simulink model "simulink"  (R2024b)
settings: Solver=ode4  StartTime=0.0  StopTime=60  FixedStep=0.005  MaxStep=0.01  MinStep=1e-06  RelTol=1e-3
values from neighbouring files (symbols this model uses):
  Cd = 0.36    [main.m]
  Cr = 0.01    [main.m]
  gear_ratio = 5    [main.m]
  initial_velocity = 0    [main.m]
  max_brake_torque = 20000    [main.m]
  track_x = track_x(:)    [main.m]    (also in plotRaceTrack.m = [x1, x2, x3, x4])
  track_y = track_y(:)    [main.m]    (also in plotRaceTrack.m = [y1, y2, y3, y4])
  v_des_straight = 15    [main.m]
  v_des_turn = 10    [main.m]
undefined symbols (not defined in the file or in its folder): carData, datBat, datMotor
libraries: slpidlib x2
settings Model: Creator=gavin  LastModifiedBy=sharj
settings SolverCC: InitialStep=1e-06

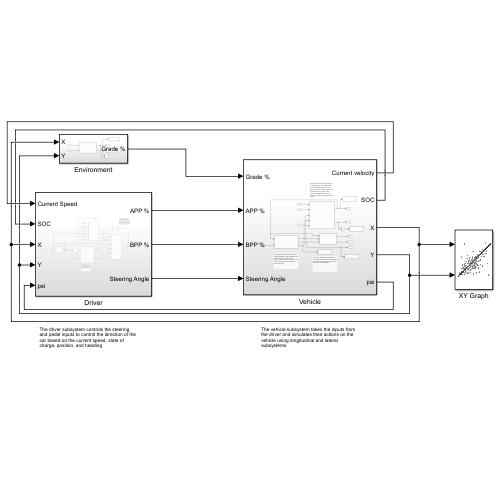
[thumbnail: Simulink's stored preview of the top-level diagram]
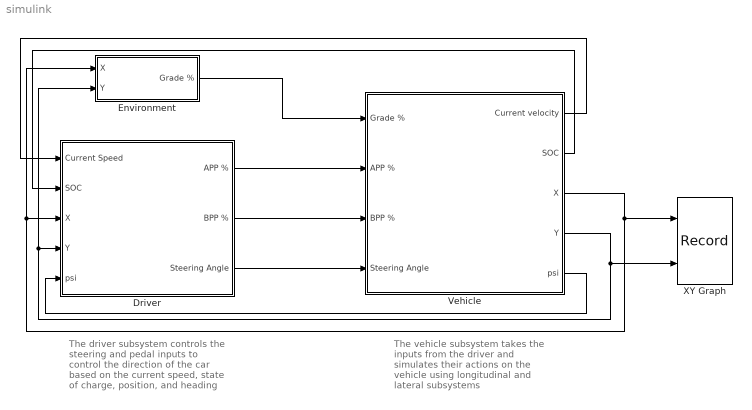
== system simulink ==
  note: The driver subsystem controls the steering and pedal inputs to control the direction of the car based on the current speed, state of charge, position, and heading
  note: The vehicle subsystem takes the inputs from the driver and simulates their actions on the vehicle using longitudinal and lateral subsystems
  Driver : Subsystem
  Environment : Subsystem
  Vehicle : Subsystem
  XY Graph : Record  FileSettingsInternal="{\"entries\":[{\"content\":{\"excelSettings\":{\"content\":{},\"type\":\"Streamout.ExcelSettings\"}},\"type\":\"Streamout.FileSettingStorage\",\"uuid\":\"\"}],\"packageUris\":[\"http:\\/\\/schema.mathworks.com\\/mf0\\/streamout_blocks\\/R2020a\"],\"version\":\"1.0\"}"  Layout=[1 1]  SignalsInternal="{\"entries\":[{\"content\":{\"signals\":[{\"content\":{\"blockPath\":[],\"dimensions\":[1],\"domain\":\"\",\"lineColor\":\"#a2142f\",\"plots\":[ 1 ],\"port\":1,\"signalID\":1,\"signalName\":\"Vehicle:3\"},\"type\":\"RecordBlkView.Signal\",\"uuid\":\"\"},{\"content\":{\"blockPath\":[],\"dimensions\":[1],\"domain\":\"\",\"lineColor\":\"#139fff\",\"plots\":[ 1 ],\"port\":2,\"signalID\":2,\"signalName\":\"Vehicle:4\"},\"type\":\"RecordBlkView.Signal\",\"uuid\":\"\"}]},\"type\":\"RecordBlkView.InputSignals\",\"uuid\":\"\"}],\"packageUris\":[\"http:\\/\\/schema.mathworks.com\\/mf0\\/streamout_blocks\\/R2020a\"],\"version\":\"1.0\"}"  VisualizationBindings="{\"xyplotplugin\":{\"info\":[{\"series\":[{\"bindingParametersList\":[{\"parameter\":\"X-Axis\",\"signalID\":1,\"signalName\":\"Vehicle:3\"},{\"parameter\":\"Y-Axis\",\"signalID\":2,\"signalName\":\"Vehicle:4\"}],\"seriesID\":0}],\"subplotID\":1}]}}"  CompatibilityTag=XY
  wires:
  Vehicle/3(X) -> XY Graph/1, Environment/1(X), Driver/3(X)
  Vehicle/4(Y) -> Environment/2(Y), Driver/4(Y), XY Graph/2
  Driver/1(APP %) -> Vehicle/2(APP %)
  Driver/2(BPP %) -> Vehicle/3(BPP %)
  Driver/3(Steering Angle) -> Vehicle/4(Steering Angle)
  Environment/1(Grade %) -> Vehicle/1(Grade %)
  Vehicle/2(SOC) -> Driver/2(SOC)
  Vehicle/1(Current velocity) -> Driver/1(Current Speed)
  Vehicle/5(psi) -> Driver/5(psi)

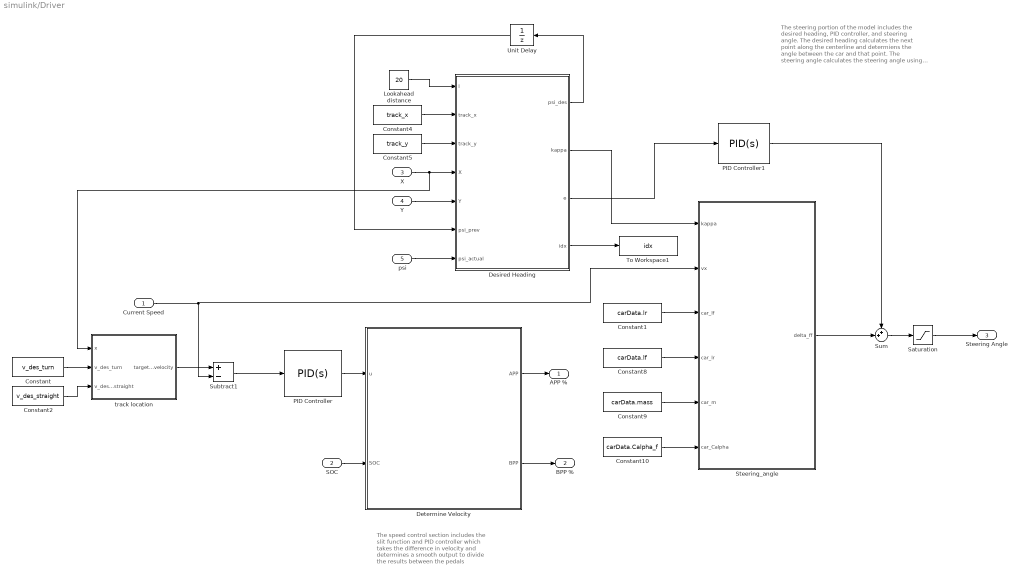
== system simulink/Driver ==
  note: The speed control section includes the slit function and PID controller which takes the difference in velocity and determines a smooth output to divide the results between the pedals
  note: The steering portion of the model includes the desired heading, PID controller, and steering angle. The desired heading calculates the next point along the centerline and determiens the angle between the car and that point. The steering angle calculates the steering angle using the feed forward method. The PID controller smooths the results and provides feedback to ensure resilience to small changes in the system.
  Current Speed : Inport
  SOC : Inport  Port=2
  X : Inport  Port=3
  Y : Inport  Port=4
  psi : Inport  Port=5
  Constant : Constant  Value=v_des_turn
  Constant1 : Constant  Value=carData.lr
  Constant10 : Constant  Value=carData.Calpha_f
  Constant2 : Constant  Value=v_des_straight
  Constant4 : Constant  Value=track_x
  Constant5 : Constant  Value=track_y
  Constant8 : Constant  Value=carData.lf
  Constant9 : Constant  Value=carData.mass
  Desired Heading : MATLAB Function  TreatAsAtomicUnit=on
  Determine Velocity : MATLAB Function  TreatAsAtomicUnit=on
  Lookahead distance : Constant  Value=20
  PID Controller : slpidlib/PID Controller  Controller=PID  Form=Parallel  TimeDomain=Continuous-time  UseExternalTs=off  SampleTime=-1  IntegratorMethod=Forward Euler  FilterMethod=Forward Euler  ControllerParametersSource=internal  P=0.9  I=0.2  UseKiTs=off  D=0  UseExternalDerivativeSource=off  N=100  UseFilter=on  TunerSelectOption=Transfer Function Based (PID Tuner App)  InitialConditionSource=internal  InitialConditionForIntegrator=0  InitialConditionForFilter=0  DifferentiatorICPrevScaledInput=0  ExternalReset=none  TrackingMode=off  Kt=1  LimitOutput=on  SatLimitsSource=internal  UpperSaturationLimit=1  LowerSaturationLimit=-1  LinearizeAsGain=on  AntiWindupMode=none  Kb=1  LimitIntegrator=off  UpperIntegratorSaturationLimit=inf  LowerIntegratorSaturationLimit=-inf  POutMin=[]  POutMax=[]  IOutMin=[]  IOutMax=[]  DOutMin=[]  DOutMax=[]  NOutMin=[]  NOutMax=[]  SumOutMin=[]  SumOutMax=[]  SaturationOutMin=[]  SaturationOutMax=[]  PParamMin=[]  PParamMax=[]  IParamMin=[]  IParamMax=[]  DParamMin=[]  DParamMax=[]  NParamMin=[]  NParamMax=[]  KbParamMin=[]  KbParamMax=[]  KtParamMin=[]  KtParamMax=[]  KbOutMin=[]  KbOutMax=[]  KtOutMin=[]  KtOutMax=[]  IntegratorOutMin=[]  IntegratorOutMax=[]  FilterOutMin=[]  FilterOutMax=[]  SumI1OutMin=[]  SumI1OutMax=[]  SumI2OutMin=[]  SumI2OutMax=[]  SumI3OutMin=[]  SumI3OutMax=[]  SumI4OutMin=[]  SumI4OutMax=[]  SumDOutMin=[]  SumDOutMax=[]  DifferentiatorOutMin=[]  DifferentiatorOutMax=[]  FilterDiffOutCoefMin=[]  FilterDiffOutCoefMax=[]  ReciprocalOutMin=[]  ReciprocalOutMax=[]  SumDenOutMin=[]  SumDenOutMax=[]  SumNumOutMin=[]  SumNumOutMax=[]  DivideOutMin=[]  DivideOutMax=[]  UdiffTsProdOutMin=[]  UdiffTsProdOutMax=[]  NTsProdOutMin=[]  NTsProdOutMax=[]  UintegralTsProdOutMin=[]  UintegralTsProdOutMax=[]  UngainTsProdOutMin=[]  UngainTsProdOutMax=[]  ClampingZeroOutDataTypeStr=Inherit: Inherit via back propagation  ClampingZeroOutMin=[]  ClampingZeroOutMax=[]  FilterDenConstantOutDataTypeStr=Inherit: Inherit via back propagation  FilterDenConstantOutMin=[]  FilterDenConstantOutMax=[]  PCopyOutDataTypeStr=Inherit: Inherit via back propagation  PCopyOutMin=[]  PCopyOutMax=[]  NCopyOutDataTypeStr=Inherit: Inherit via back propagation  NCopyOutMin=[]  NCopyOutMax=[]  IntegratorContinuousStateAttributes=''  IntegratorStateMustResolveToSignalObject=off  IntegratorRTWStateStorageClass=Auto  FilterContinuousStateAttributes=''  FilterStateMustResolveToSignalObject=off  FilterRTWStateStorageClass=Auto  ParallelPVariant=InternalParameters  IdealPVariant=Disabled  IVariant=InternalParameters  DVariant=InternalParameters  IntegratorVariant=Continuous  SatVariant=Disabled  AWVariant=Passthrough  PCopyVariant=Disabled  TRVariant=Disabled  FdbkBlocksVariant=Forward  IdealPFdbkVariant=Disabled  SatFdbkVariant=Disabled  DerivativeFilterVariant=ContFilter  NVariant=InternalParameters  NCopyVariant=Disabled  FilterICVariant=InternalICsFilter  IntegratorICVariant=InternalICs  ExternalResetVariant=Disabled  TRSumVariant=Passthrough  SumFdbkVariant=Disabled  SumVariant=Sum_PID  TsampFilterVariant=InternalTs  TsampNgainVariant=Passthrough  TsampIntegralVariant=Passthrough  ExternalSaturationOutDataTypeStr=Inherit: Same as second input  DerivativeSourceVariant=ErrorSignal  PreIntVariant=InternalPreInt
  PID Controller1 : slpidlib/PID Controller  Controller=PID  Form=Parallel  TimeDomain=Continuous-time  UseExternalTs=off  SampleTime=-1  IntegratorMethod=Forward Euler  FilterMethod=Forward Euler  ControllerParametersSource=internal  P=1  I=1  UseKiTs=off  D=0  UseExternalDerivativeSource=off  N=100  UseFilter=on  TunerSelectOption=Transfer Function Based (PID Tuner App)  InitialConditionSource=internal  InitialConditionForIntegrator=0  InitialConditionForFilter=0  DifferentiatorICPrevScaledInput=0  ExternalReset=none  TrackingMode=off  Kt=1  LimitOutput=off  SatLimitsSource=internal  UpperSaturationLimit=inf  LowerSaturationLimit=-inf  LinearizeAsGain=on  AntiWindupMode=none  Kb=1  LimitIntegrator=off  UpperIntegratorSaturationLimit=inf  LowerIntegratorSaturationLimit=-inf  POutMin=[]  POutMax=[]  IOutMin=[]  IOutMax=[]  DOutMin=[]  DOutMax=[]  NOutMin=[]  NOutMax=[]  SumOutMin=[]  SumOutMax=[]  SaturationOutMin=[]  SaturationOutMax=[]  PParamMin=[]  PParamMax=[]  IParamMin=[]  IParamMax=[]  DParamMin=[]  DParamMax=[]  NParamMin=[]  NParamMax=[]  KbParamMin=[]  KbParamMax=[]  KtParamMin=[]  KtParamMax=[]  KbOutMin=[]  KbOutMax=[]  KtOutMin=[]  KtOutMax=[]  IntegratorOutMin=[]  IntegratorOutMax=[]  FilterOutMin=[]  FilterOutMax=[]  SumI1OutMin=[]  SumI1OutMax=[]  SumI2OutMin=[]  SumI2OutMax=[]  SumI3OutMin=[]  SumI3OutMax=[]  SumI4OutMin=[]  SumI4OutMax=[]  SumDOutMin=[]  SumDOutMax=[]  DifferentiatorOutMin=[]  DifferentiatorOutMax=[]  FilterDiffOutCoefMin=[]  FilterDiffOutCoefMax=[]  ReciprocalOutMin=[]  ReciprocalOutMax=[]  SumDenOutMin=[]  SumDenOutMax=[]  SumNumOutMin=[]  SumNumOutMax=[]  DivideOutMin=[]  DivideOutMax=[]  UdiffTsProdOutMin=[]  UdiffTsProdOutMax=[]  NTsProdOutMin=[]  NTsProdOutMax=[]  UintegralTsProdOutMin=[]  UintegralTsProdOutMax=[]  UngainTsProdOutMin=[]  UngainTsProdOutMax=[]  ClampingZeroOutDataTypeStr=Inherit: Inherit via back propagation  ClampingZeroOutMin=[]  ClampingZeroOutMax=[]  FilterDenConstantOutDataTypeStr=Inherit: Inherit via back propagation  FilterDenConstantOutMin=[]  FilterDenConstantOutMax=[]  PCopyOutDataTypeStr=Inherit: Inherit via back propagation  PCopyOutMin=[]  PCopyOutMax=[]  NCopyOutDataTypeStr=Inherit: Inherit via back propagation  NCopyOutMin=[]  NCopyOutMax=[]  IntegratorContinuousStateAttributes=''  IntegratorStateMustResolveToSignalObject=off  IntegratorRTWStateStorageClass=Auto  FilterContinuousStateAttributes=''  FilterStateMustResolveToSignalObject=off  FilterRTWStateStorageClass=Auto  ParallelPVariant=InternalParameters  IdealPVariant=Disabled  IVariant=InternalParameters  DVariant=InternalParameters  IntegratorVariant=Continuous  SatVariant=Disabled  AWVariant=Passthrough  PCopyVariant=Disabled  TRVariant=Disabled  FdbkBlocksVariant=Forward  IdealPFdbkVariant=Disabled  SatFdbkVariant=Disabled  DerivativeFilterVariant=ContFilter  NVariant=InternalParameters  NCopyVariant=Disabled  FilterICVariant=InternalICsFilter  IntegratorICVariant=InternalICs  ExternalResetVariant=Disabled  TRSumVariant=Passthrough  SumFdbkVariant=Disabled  SumVariant=Sum_PID  TsampFilterVariant=InternalTs  TsampNgainVariant=Passthrough  TsampIntegralVariant=Passthrough  ExternalSaturationOutDataTypeStr=Inherit: Same as second input  DerivativeSourceVariant=ErrorSignal  PreIntVariant=InternalPreInt
  Saturation : Saturate
  Steering_angle : MATLAB Function  TreatAsAtomicUnit=on
  Subtract1 : Sum  Inputs=+-
  Sum : Sum  Inputs=++|
  To Workspace1 : ToWorkspace  VariableName=idx  SaveFormat=Timeseries  SampleTime=-1
  Unit Delay : UnitDelay  SampleTime=-1  HasFrameUpgradeWarning=on
  track location : MATLAB Function  TreatAsAtomicUnit=on
  APP % : Outport
  BPP % : Outport  Port=2
  Steering Angle : Outport  Port=3
  wires:
  Constant1/1 -> Steering_angle/3(car_lf)
  Lookahead distance/1 -> Desired Heading/1(l)
  Desired Heading/1(psi_des) -> Unit Delay/1
  Desired Heading/2(kappa) -> Steering_angle/1(kappa)
  Determine Velocity/1(APP) -> APP %/1
  Determine Velocity/2(BPP) -> BPP %/1
  Unit Delay/1 -> Desired Heading/6(psi_prev)
  Constant5/1 -> Desired Heading/3(track_y)
  Constant4/1 -> Desired Heading/2(track_x)
  X/1 -> track location/1(x), Desired Heading/4(X)
  Y/1 -> Desired Heading/5(Y)
  SOC/1 -> Determine Velocity/2(SOC)
  Constant10/1 -> Steering_angle/6(car_Calpha)
  Constant9/1 -> Steering_angle/5(car_m)
  Constant8/1 -> Steering_angle/4(car_lr)
  Subtract1/1 -> PID Controller/1
  Current Speed/1 -> Subtract1/2, Steering_angle/2(vx)
  PID Controller/1 -> Determine Velocity/1(u)
  Desired Heading/3(e) -> PID Controller1/1
  PID Controller1/1 -> Sum/1
  Sum/1 -> Saturation/1
  psi/1 -> Desired Heading/7(psi_actual)
  Desired Heading/4(idx) -> To Workspace1/1
  Steering_angle/1(delta_ff) -> Sum/2
  Saturation/1 -> Steering Angle/1
  Constant2/1 -> track location/3(v_des_straight)
  Constant/1 -> track location/2(v_des_turn)
  track location/1(target_velocity) -> Subtract1/1

== system simulink/Environment ==
  X : Inport
  Y : Inport  Port=2
  MATLAB Function : MATLAB Function  TreatAsAtomicUnit=on
  To Workspace : ToWorkspace  VariableName=grade  SaveFormat=Timeseries  SampleTime=-1
  To Workspace1 : ToWorkspace  VariableName=height  SaveFormat=Timeseries  SampleTime=-1
  height and grade scope : Scope  NumInputPorts=2
  Grade % : Outport
  wires:
  Y/1 -> MATLAB Function/2(y)
  X/1 -> MATLAB Function/1(x)
  MATLAB Function/2(height) -> height and grade scope/1, To Workspace1/1
  MATLAB Function/1(gradePct) -> height and grade scope/2, To Workspace/1, Grade %/1

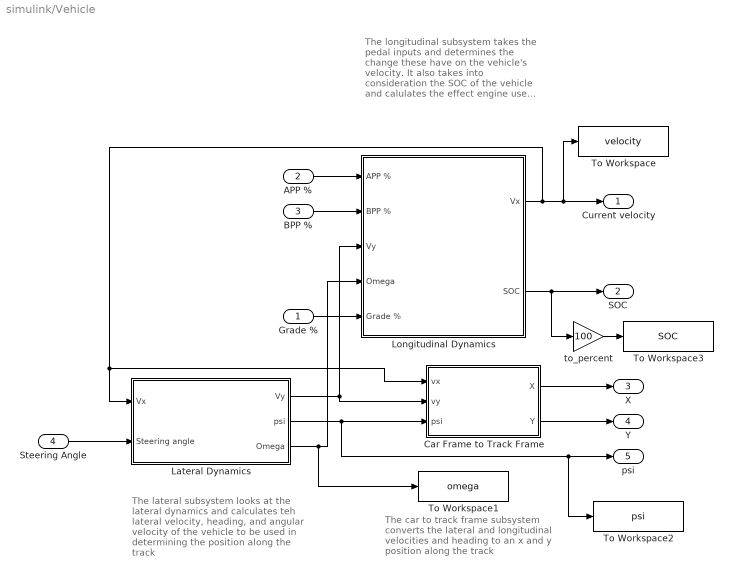
== system simulink/Vehicle ==
  note: The lateral subsystem looks at the lateral dynamics and calculates teh lateral velocity, heading, and angular velocity of the vehicle to be used in determining the position along the track
  note: The car to track frame subsystem converts the lateral and longitudinal velocities and heading to an x and y position along the track
  note: The longitudinal subsystem takes the pedal inputs and determines the change these have on the vehicle's velocity. It also takes into consideration the SOC of the vehicle and calulates the effect engine use and regen braking have on this.
  Grade % : Inport
  APP % : Inport  Port=2
  BPP % : Inport  Port=3
  Steering Angle : Inport  Port=4
  Car Frame to Track Frame : Subsystem
  Lateral Dynamics : Subsystem
  Longitudinal Dynamics : Subsystem
  To Workspace : ToWorkspace  VariableName=velocity  SaveFormat=Timeseries  SampleTime=-1
  To Workspace1 : ToWorkspace  VariableName=omega  SaveFormat=Timeseries  SampleTime=-1
  To Workspace2 : ToWorkspace  VariableName=psi  SaveFormat=Timeseries  SampleTime=-1
  To Workspace3 : ToWorkspace  VariableName=SOC  SaveFormat=Timeseries  SampleTime=-1
  to_percent : Gain  Gain=100
  Current velocity : Outport
  SOC : Outport  Port=2
  X : Outport  Port=3
  Y : Outport  Port=4
  psi : Outport  Port=5
  wires:
  Longitudinal Dynamics/1(Vx) -> To Workspace/1, Current velocity/1, Car Frame to Track Frame/1(vx), Lateral Dynamics/1(Vx)
  Longitudinal Dynamics/2(SOC) -> to_percent/1, SOC/1
  Grade %/1 -> Longitudinal Dynamics/5(Grade %)
  APP %/1 -> Longitudinal Dynamics/1(APP %)
  BPP %/1 -> Longitudinal Dynamics/2(BPP %)
  Steering Angle/1 -> Lateral Dynamics/2(Steering angle)
  Lateral Dynamics/1(Vy) -> Car Frame to Track Frame/2(vy), Longitudinal Dynamics/3(Vy)
  Lateral Dynamics/3(Omega) -> To Workspace1/1, Longitudinal Dynamics/4(Omega)
  Car Frame to Track Frame/1(X) -> X/1
  Car Frame to Track Frame/2(Y) -> Y/1
  Lateral Dynamics/2(psi) -> To Workspace2/1, psi/1, Car Frame to Track Frame/3(psi)
  to_percent/1 -> To Workspace3/1

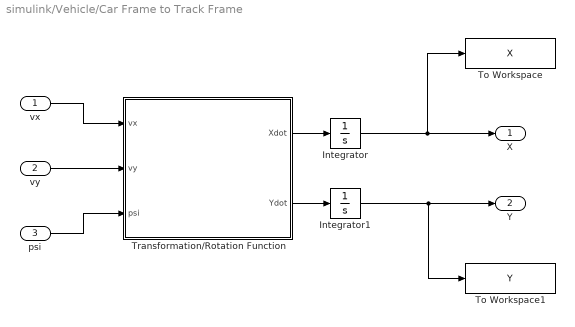
== system simulink/Vehicle/Car Frame to Track Frame ==
  vx : Inport
  vy : Inport  Port=2
  psi : Inport  Port=3
  Integrator : Integrator
  Integrator1 : Integrator
  To Workspace : ToWorkspace  VariableName=X  SaveFormat=Timeseries  SampleTime=-1
  To Workspace1 : ToWorkspace  VariableName=Y  SaveFormat=Timeseries  SampleTime=-1
  Transformation/Rotation Function : MATLAB Function  TreatAsAtomicUnit=on
  X : Outport
  Y : Outport  Port=2
  wires:
  vy/1 -> Transformation/Rotation Function/2(vy)
  Transformation/Rotation Function/2(Ydot) -> Integrator1/1
  psi/1 -> Transformation/Rotation Function/3(psi)
  vx/1 -> Transformation/Rotation Function/1(vx)
  Integrator/1 -> To Workspace/1, X/1
  Transformation/Rotation Function/1(Xdot) -> Integrator/1
  Integrator1/1 -> To Workspace1/1, Y/1

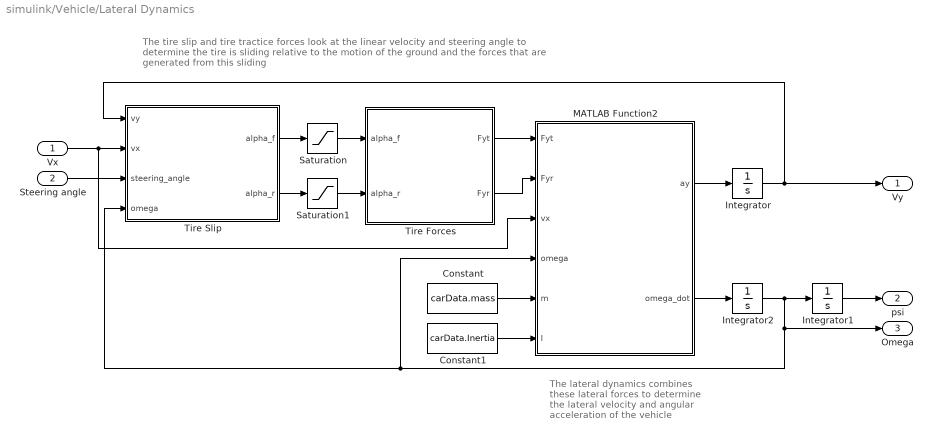
== system simulink/Vehicle/Lateral Dynamics ==
  note: The tire slip and tire tractice forces look at the linear velocity and steering angle to determine the tire is sliding relative to the motion of the ground and the forces that are generated from this sliding
  note: The lateral dynamics combines these lateral forces to determine the lateral velocity and angular acceleration of the vehicle
  Vx : Inport
  Steering angle : Inport  Port=2
  Constant : Constant  Value=carData.mass
  Constant1 : Constant  Value=carData.Inertia
  Integrator : Integrator
  Integrator1 : Integrator
  Integrator2 : Integrator
  MATLAB Function2 : MATLAB Function  TreatAsAtomicUnit=on
  Saturation : Saturate  UpperLimit=0.2  LowerLimit=-0.2
  Saturation1 : Saturate  UpperLimit=0.2  LowerLimit=-0.2
  Tire Forces : MATLAB Function  TreatAsAtomicUnit=on
  Tire Slip : MATLAB Function  TreatAsAtomicUnit=on
  Vy : Outport
  psi : Outport  Port=2
  Omega : Outport  Port=3
  wires:
  Vx/1 -> MATLAB Function2/3(vx), Tire Slip/2(vx)
  Steering angle/1 -> Tire Slip/3(steering_angle)
  Tire Forces/1(Fyt) -> MATLAB Function2/1(Fyt)
  Tire Forces/2(Fyr) -> MATLAB Function2/2(Fyr)
  MATLAB Function2/2(omega_dot) -> Integrator2/1
  Integrator2/1 -> Integrator1/1, Omega/1, MATLAB Function2/4(omega), Tire Slip/4(omega)
  Integrator1/1 -> psi/1
  Integrator/1 -> Tire Slip/1(vy), Vy/1
  MATLAB Function2/1(ay) -> Integrator/1
  Tire Slip/1(alpha_f) -> Saturation/1
  Saturation/1 -> Tire Forces/1(alpha_f)
  Tire Slip/2(alpha_r) -> Saturation1/1
  Saturation1/1 -> Tire Forces/2(alpha_r)
  Constant/1 -> MATLAB Function2/5(m)
  Constant1/1 -> MATLAB Function2/6(I)

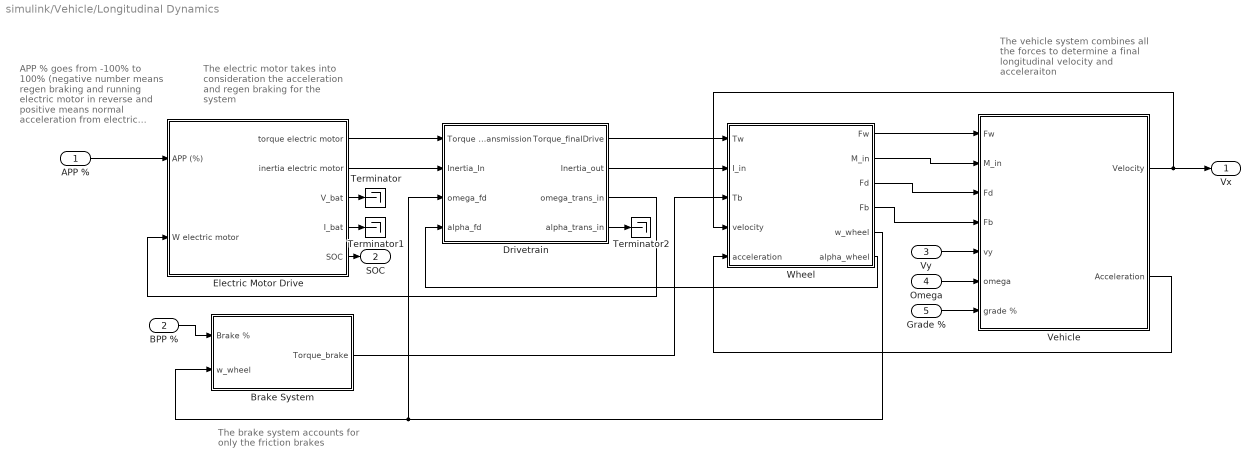
== system simulink/Vehicle/Longitudinal Dynamics ==
  note: APP % goes from -100% to 100% (negative number means regen braking and running electric motor in reverse and positive means normal acceleration from electric motor)
  note: The electric motor takes into consideration the acceleration and regen braking for the system
  note: The brake system accounts for only the friction brakes
  note: The vehicle system combines all the forces to determine a final longitudinal velocity and acceleraiton
  APP % : Inport
  BPP % : Inport  Port=2
  Vy : Inport  Port=3
  Omega : Inport  Port=4
  Grade % : Inport  Port=5
  Brake System : Subsystem
  Drivetrain : Subsystem
  Electric Motor Drive : Subsystem
  Terminator : Terminator
  Terminator1 : Terminator
  Terminator2 : Terminator
  Vehicle : Subsystem
  Wheel : Subsystem
  Vx : Outport
  SOC : Outport  Port=2
  wires:
  Vehicle/1(Velocity) -> Wheel/4(velocity), Vx/1
  Electric Motor Drive/5(SOC) -> SOC/1
  APP %/1 -> Electric Motor Drive/1(APP (%))
  BPP %/1 -> Brake System/1(Brake %)
  Vy/1 -> Vehicle/5(vy)
  Omega/1 -> Vehicle/6(omega)
  Grade %/1 -> Vehicle/7(grade %)
  Electric Motor Drive/3(V_bat) -> Terminator/1
  Electric Motor Drive/4(I_bat) -> Terminator1/1
  Drivetrain/4(alpha_trans_in) -> Terminator2/1
  Electric Motor Drive/1(torque electric motor) -> Drivetrain/1(Torque Transmission)
  Electric Motor Drive/2(inertia electric motor) -> Drivetrain/2(Inertia_In)
  Wheel/5(w_wheel) -> Brake System/2(w_wheel), Drivetrain/3(omega_fd)
  Wheel/6(alpha_wheel) -> Drivetrain/4(alpha_fd)
  Drivetrain/1(Torque_finalDrive) -> Wheel/1(Tw)
  Drivetrain/2(Inertia_out) -> Wheel/2(I_in)
  Drivetrain/3(omega_trans_in) -> Electric Motor Drive/2(W electric motor)
  Brake System/1(Torque_brake) -> Wheel/3(Tb)
  Wheel/1(Fw) -> Vehicle/1(Fw)
  Wheel/2(M_in) -> Vehicle/2(M_in)
  Vehicle/2(Acceleration) -> Wheel/5(acceleration)
  Wheel/3(Fd) -> Vehicle/3(Fd)
  Wheel/4(Fb) -> Vehicle/4(Fb)

== system simulink/Vehicle/Longitudinal Dynamics/Brake System ==
  Brake % : Inport
  w_wheel : Inport  Port=2
  Constant : Constant  Value=max_brake_torque
  MATLAB Function : MATLAB Function  TreatAsAtomicUnit=on
  Torque_brake : Outport
  wires:
  Brake %/1 -> MATLAB Function/1(BBcmd)
  w_wheel/1 -> MATLAB Function/3(w_wheel)
  MATLAB Function/1(Tb) -> Torque_brake/1
  Constant/1 -> MATLAB Function/2(Tbcap)

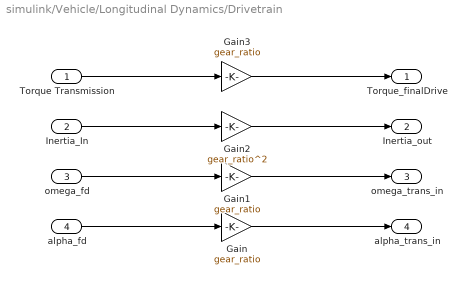
== system simulink/Vehicle/Longitudinal Dynamics/Drivetrain ==
  Torque Transmission : Inport
  Inertia_In : Inport  Port=2
  omega_fd : Inport  Port=3
  alpha_fd : Inport  Port=4
  Gain : Gain  Gain=gear_ratio
  Gain1 : Gain  Gain=gear_ratio
  Gain2 : Gain  Gain=gear_ratio^2
  Gain3 : Gain  Gain=gear_ratio
  Torque_finalDrive : Outport
  Inertia_out : Outport  Port=2
  omega_trans_in : Outport  Port=3
  alpha_trans_in : Outport  Port=4
  wires:
  Torque Transmission/1 -> Gain3/1
  Gain3/1 -> Torque_finalDrive/1
  Inertia_In/1 -> Gain2/1
  Gain2/1 -> Inertia_out/1
  Gain1/1 -> omega_trans_in/1
  omega_fd/1 -> Gain1/1
  Gain/1 -> alpha_trans_in/1
  alpha_fd/1 -> Gain/1

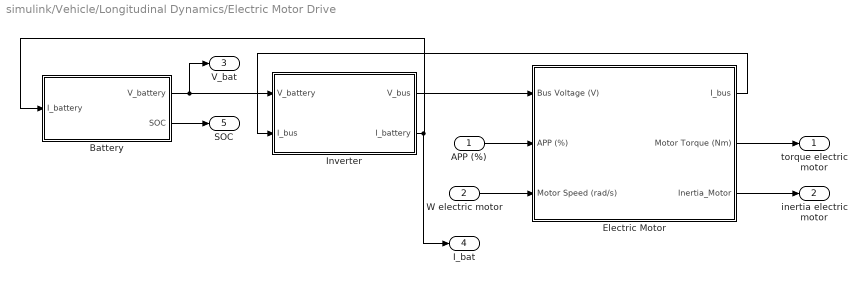
== system simulink/Vehicle/Longitudinal Dynamics/Electric Motor Drive ==
  APP (%) : Inport
  W electric motor : Inport  Port=2
  Battery : Subsystem
  Electric Motor : Subsystem
  Inverter : Subsystem
  torque electric motor : Outport
  inertia electric motor : Outport  Port=2
  V_bat : Outport  Port=3
  I_bat : Outport  Port=4
  SOC : Outport  Port=5
  wires:
  Battery/1(V_battery) -> Inverter/1(V_battery), V_bat/1
  Battery/2(SOC) -> SOC/1
  Inverter/1(V_bus) -> Electric Motor/1(Bus Voltage (V))
  W electric motor/1 -> Electric Motor/3(Motor Speed (rad/s))
  APP (%)/1 -> Electric Motor/2(APP (%))
  Electric Motor/1(I_bus) -> Inverter/2(I_bus)
  Inverter/2(I_battery) -> I_bat/1, Battery/1(I_battery)
  Electric Motor/3(Inertia_Motor) -> inertia electric motor/1
  Electric Motor/2(Motor Torque (Nm)) -> torque electric motor/1

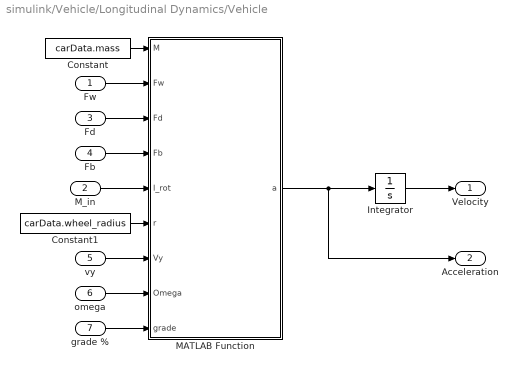
== system simulink/Vehicle/Longitudinal Dynamics/Vehicle ==
  Fw : Inport
  M_in : Inport  Port=2
  Fd : Inport  Port=3
  Fb : Inport  Port=4
  vy : Inport  Port=5
  omega : Inport  Port=6
  grade % : Inport  Port=7
  Constant : Constant  Value=carData.mass
  Constant1 : Constant  Value=carData.wheel_radius
  Integrator : Integrator  InitialCondition=initial_velocity
  MATLAB Function : MATLAB Function  TreatAsAtomicUnit=on
  Velocity : Outport
  Acceleration : Outport  Port=2
  wires:
  grade %/1 -> MATLAB Function/9(grade)
  vy/1 -> MATLAB Function/7(Vy)
  M_in/1 -> MATLAB Function/5(I_rot)
  Fw/1 -> MATLAB Function/2(Fw)
  Integrator/1 -> Velocity/1
  Constant/1 -> MATLAB Function/1(M)
  Fb/1 -> MATLAB Function/4(Fb)
  Fd/1 -> MATLAB Function/3(Fd)
  Constant1/1 -> MATLAB Function/6(r)
  omega/1 -> MATLAB Function/8(Omega)
  MATLAB Function/1(a) -> Integrator/1, Acceleration/1

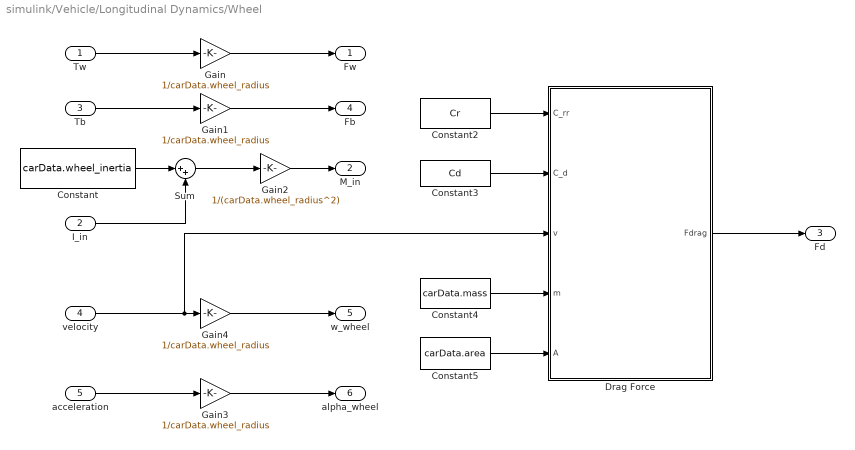
== system simulink/Vehicle/Longitudinal Dynamics/Wheel ==
  Tw : Inport
  I_in : Inport  Port=2
  Tb : Inport  Port=3
  velocity : Inport  Port=4
  acceleration : Inport  Port=5
  Constant : Constant  Value=carData.wheel_inertia
  Constant2 : Constant  Value=Cr
  Constant3 : Constant  Value=Cd
  Constant4 : Constant  Value=carData.mass
  Constant5 : Constant  Value=carData.area
  Drag Force : MATLAB Function  TreatAsAtomicUnit=on
  Gain{,1,3..4} (4 alike) : Gain  Gain=1/carData.wheel_radius
  Gain2 : Gain  Gain=1/(carData.wheel_radius^2)
  Sum : Sum  Inputs=|++
  Fw : Outport
  M_in : Outport  Port=2
  Fd : Outport  Port=3
  Fb : Outport  Port=4
  w_wheel : Outport  Port=5
  alpha_wheel : Outport  Port=6
  wires:
  Tw/1 -> Gain/1
  Gain/1 -> Fw/1
  Tb/1 -> Gain1/1
  Gain1/1 -> Fb/1
  Constant/1 -> Sum/1
  I_in/1 -> Sum/2
  Sum/1 -> Gain2/1
  Gain2/1 -> M_in/1
  velocity/1 -> Drag Force/3(v), Gain4/1
  Gain4/1 -> w_wheel/1
  Gain3/1 -> alpha_wheel/1
  acceleration/1 -> Gain3/1
  Drag Force/1(Fdrag) -> Fd/1
  Constant2/1 -> Drag Force/1(C_rr)
  Constant3/1 -> Drag Force/2(C_d)
  Constant4/1 -> Drag Force/4(m)
  Constant5/1 -> Drag Force/5(A)

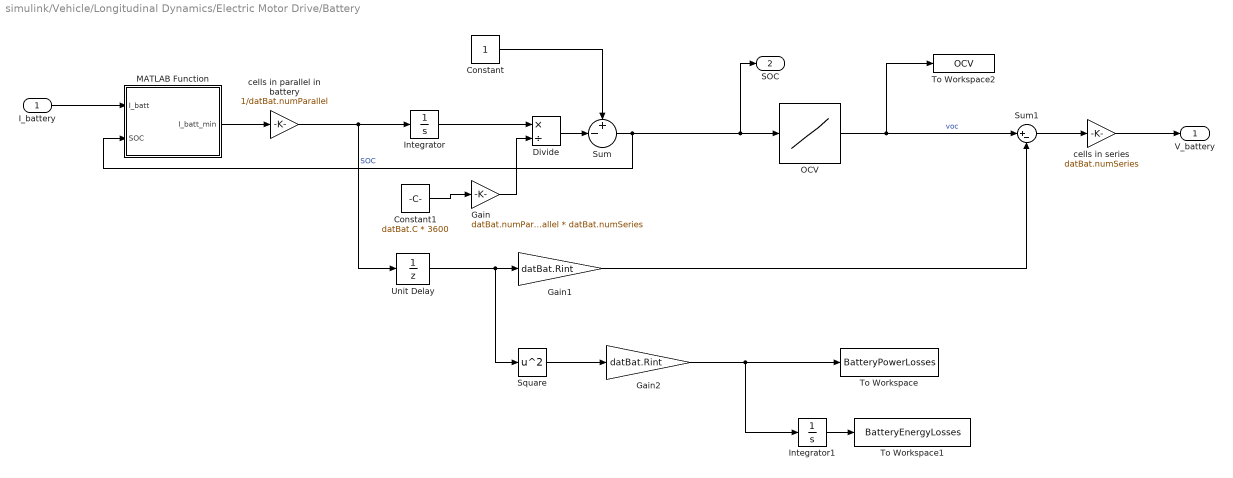
== system simulink/Vehicle/Longitudinal Dynamics/Electric Motor Drive/Battery ==
  I_battery : Inport
  Constant : Constant
  Constant1 : Constant  Value=datBat.C * 3600
  Divide : Product  Inputs=*/
  Gain : Gain  Gain=datBat.numParallel * datBat.numSeries
  Gain1 : Gain  Gain=datBat.Rint
  Gain2 : Gain  Gain=datBat.Rint
  Integrator : Integrator
  Integrator1 : Integrator
  MATLAB Function : MATLAB Function  TreatAsAtomicUnit=on
  OCV : Lookup_n-D  NumberOfTableDimensions=1  BreakpointsForDimension1=datBat.SOC  Table=datBat.OCV  InternalRulePriority=Speed  RndMeth=Simplest
  Square : Math  Operator=square
  Sum : Sum  Inputs=+-|
  Sum1 : Sum  Inputs=|+-
  To Workspace : ToWorkspace  VariableName=BatteryPowerLosses  SaveFormat=Timeseries  SampleTime=-1
  To Workspace1 : ToWorkspace  VariableName=BatteryEnergyLosses  SaveFormat=Timeseries  SampleTime=-1
  To Workspace2 : ToWorkspace  VariableName=OCV  SaveFormat=Timeseries  SampleTime=-1
  Unit Delay : UnitDelay  SampleTime=-1  HasFrameUpgradeWarning=on
  cells in parallel in battery : Gain  Gain=1/datBat.numParallel
  cells in series : Gain  Gain=datBat.numSeries
  V_battery : Outport
  SOC : Outport  Port=2
  wires:
  I_battery/1 -> MATLAB Function/1(I_batt)
  MATLAB Function/1(I_batt_min) -> cells in parallel in battery/1
  Constant/1 -> Sum/1
  Constant1/1 -> Gain/1
  Gain/1 -> Divide/2
  Integrator/1 -> Divide/1
  Divide/1 -> Sum/2
  cells in parallel in battery/1 -> Unit Delay/1, Integrator/1
  Unit Delay/1 -> Square/1, Gain1/1
  Square/1 -> Gain2/1
  Integrator1/1 -> To Workspace1/1
  Gain2/1 -> To Workspace/1, Integrator1/1
  Sum/1 -> MATLAB Function/2(SOC), SOC/1, OCV/1  "SOC"
  OCV/1 -> To Workspace2/1, Sum1/1  "voc"
  Gain1/1 -> Sum1/2
  Sum1/1 -> cells in series/1
  cells in series/1 -> V_battery/1

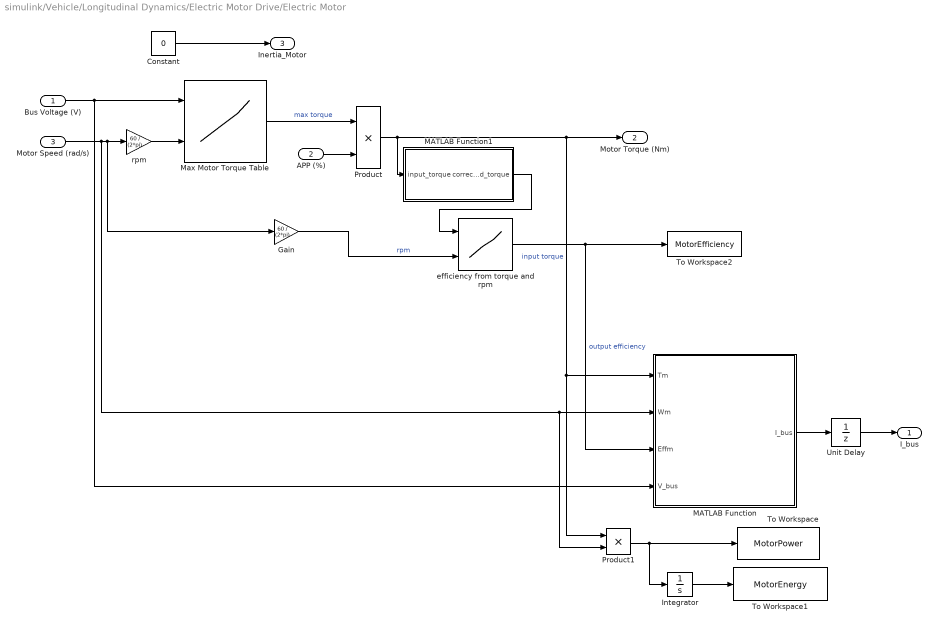
== system simulink/Vehicle/Longitudinal Dynamics/Electric Motor Drive/Electric Motor ==
  Bus Voltage (V) : Inport
  APP (%) : Inport  Port=2
  Motor Speed (rad/s) : Inport  Port=3
  Constant : Constant  Value=0
  Gain : Gain  Gain=60 / (2*pi)
  Integrator : Integrator
  MATLAB Function : MATLAB Function  TreatAsAtomicUnit=on
  MATLAB Function1 : MATLAB Function  TreatAsAtomicUnit=on
  Max Motor Torque Table : Lookup_n-D  BreakpointsForDimension1=datMotor.vbus  BreakpointsForDimension2=datMotor.rpm  Table=datMotor.maxtorque  InternalRulePriority=Speed  RndMeth=Simplest
      settings: InputPortMap=u0,u1
  Product : Product
  Product1 : Product
  To Workspace : ToWorkspace  VariableName=MotorPower  SaveFormat=Timeseries  SampleTime=-1
  To Workspace1 : ToWorkspace  VariableName=MotorEnergy  SaveFormat=Timeseries  SampleTime=-1
  To Workspace2 : ToWorkspace  VariableName=MotorEfficiency  SaveFormat=Timeseries  SampleTime=-1
  Unit Delay : UnitDelay  SampleTime=-1  HasFrameUpgradeWarning=on
  efficiency from torque and rpm : Lookup_n-D  BreakpointsForDimension1=datMotor.eta_torque  BreakpointsForDimension2=datMotor.eta_speed  Table=datMotor.eta_val  InternalRulePriority=Speed  RndMeth=Simplest
      settings: InputPortMap=u0,u1
  rpm : Gain  Gain=60 / (2*pi)
  I_bus : Outport
  Motor Torque (Nm) : Outport  Port=2
  Inertia_Motor : Outport  Port=3
  wires:
  efficiency from torque and rpm/1 -> MATLAB Function/3(Effm), To Workspace2/1  "output efficiency"
  Product/1 -> MATLAB Function1/1(input_torque), Product1/1, MATLAB Function/1(Tm), Motor Torque (Nm)/1  "input torque"
  Bus Voltage (V)/1 -> MATLAB Function/4(V_bus), Max Motor Torque Table/1
  Motor Speed (rad/s)/1 -> Product1/2, MATLAB Function/2(Wm), Gain/1, rpm/1
  rpm/1 -> Max Motor Torque Table/2
  Max Motor Torque Table/1 -> Product/1  "max torque"
  APP (%)/1 -> Product/2
  Gain/1 -> efficiency from torque and rpm/2  "rpm"
  Unit Delay/1 -> I_bus/1
  MATLAB Function/1(I_bus) -> Unit Delay/1
  Product1/1 -> To Workspace/1, Integrator/1
  Integrator/1 -> To Workspace1/1
  Constant/1 -> Inertia_Motor/1
  MATLAB Function1/1(corrected_torque) -> efficiency from torque and rpm/1

== system simulink/Vehicle/Longitudinal Dynamics/Electric Motor Drive/Inverter ==
  V_battery : Inport
  I_bus : Inport  Port=2
  Inverter Efficiency : Constant  Value=0.95
  MATLAB Function : MATLAB Function  TreatAsAtomicUnit=on
  V_bus : Outport
  I_battery : Outport  Port=2
  wires:
  MATLAB Function/1(V_bus) -> V_bus/1
  MATLAB Function/2(I_bat) -> I_battery/1
  V_battery/1 -> MATLAB Function/1(V_bat)
  Inverter Efficiency/1 -> MATLAB Function/2(Eff_I)
  I_bus/1 -> MATLAB Function/3(I_bus)

== matlab function simulink/Driver/Determine Velocity ==
  data: u input; APP output; BPP output; SOC input
function [APP, BPP] = split_cmd(u, SOC)
% Inputs:
%   u   – PID output [-1 - +1]
%   SOC – battery state of charge (0 - 1)
%
% Outputs:
%   APP – accelerator/regeneration pedal % (–100 - +100)
%   BPP – friction brake pedal %           (0 - 100)

  SOC_max = 0.95;  % above this, no regen

  % clamp the command
  u = max(min(u, 1), -1);

  if u >= 0 % accelerating
    APP = u * 100;   % 0…+100%
    BPP = 0;
  else % braking
    brake_frac = min(-u, 1);              
    regen_frac = max(0, 1 - SOC/SOC_max); 
    regen_frac = min(regen_frac, 1);      

    % allocate between regen (negative APP) and friction (BPP)
    APP = - regen_frac * brake_frac;       
    BPP =   (1 - regen_frac) * brake_frac; 
  end

  % safety clamp
  APP = max(min(APP,  1), -1);
  BPP = max(min(BPP,  1),   0);
end

== matlab function simulink/Driver/Steering_angle ==
  data: delta_ff output; kappa input; vx input; car_lf input; car_lr input; car_m input; car_Calpha input
function delta_ff = feedforwardSteering(kappa, vx, car_lf, car_lr, car_m, car_Calpha)
% Compute the steady-state feed-forward steering angle.

  wheelbase = car_lf + car_lr;
  
  delta_ff = atan( wheelbase * kappa );

  % clamp tiny angles
  if abs(delta_ff) < deg2rad(0.1)
    delta_ff = 0;
  end
end

== matlab function simulink/Driver/Desired Heading ==
  settings: updateMethod=DISCRETE
  data: l input; psi_des output; track_x input; track_y input; X input; Y input; psi_prev input; kappa output; e output; psi_actual input; idx output
function [psi_des, kappa, e, idx] = purePursuitLookAhead(l, track_x, track_y, X, Y, psi_prev, psi_actual)
% Compute desired heading psi_des, signed curvature kappa, signed lateral
% error e, and look-ahead index idx for pure‐pursuit feed-forward.

  track_x = track_x(:);
  track_y = track_y(:);
  N       = numel(track_x);

  % search for the closest point along the centerline
  persistent lastIdx
  if isempty(lastIdx), lastIdx = 1; end
  W = 10;  % search ±10 points around previous
  i1 = max(1,   lastIdx - W);
  i2 = min(N, lastIdx + W);
  [~, rel] = min( (track_x(i1:i2)-X).^2 + (track_y(i1:i2)-Y).^2 );
  idx = i1 + rel - 1;
  lastIdx = idx;

  % determine the index of the lookahead point
  step = round(l);
  l_idx = idx + step;
  if l_idx > N, l_idx = l_idx - N;
  elseif l_idx < 1, l_idx = l_idx + N; end

  % calculate the desired heading
  psi_des = atan2(track_y(l_idx)-Y, track_x(l_idx)-X);
  psi_des = wrapToPi(psi_des);

  % calculate the curvature
  dx  = gradient(track_x);
  dy  = gradient(track_y);
  ddx = gradient(dx);
  ddy = gradient(dy);
  num = dx(idx)*ddy(idx) - dy(idx)*ddx(idx);
  den = ( dx(idx)^2 + dy(idx)^2 )^(3/2);
  kappa = num/den;
  % clamp for numerical noise
  if abs(kappa) < 1e-4
    kappa = 0;
  end

  % calculate the cross-track error
  t = [dx(idx); dy(idx)];
  t = t / norm(t);
  n = [-t(2); t(1)];             
  errVec = [X - track_x(idx); Y - track_y(idx)];
  e = n' * errVec;              
end

== matlab function simulink/Vehicle/Longitudinal Dynamics/Electric Motor Drive/Battery/MATLAB Function ==
  data: I_batt input; I_batt_min output; SOC input
function I_batt_min = fcn(I_batt, SOC)
    if SOC <= 0.1
        I_batt_min = 0;
    else
        I_batt_min = I_batt;
    end
end

== matlab function simulink/Vehicle/Longitudinal Dynamics/Electric Motor Drive/Electric Motor/MATLAB Function ==
  data: Tm input; I_bus output; Wm input; Effm input; V_bus input
function I_bus = fcn(Tm, Wm, Effm, V_bus)
    % Mechanical power (element‑wise)
    Pm = Tm .* Wm;
    
    % Sign of Pm, with tiny offset (element‑wise)
    sgn_m = (Pm + 1e-7) ./ (abs(Pm) + 1e-7) + 0.001;
    
    % Ensure Effm is strictly positive to avoid negative base errors
    Effm_pos = abs(Effm) + eps;  
    
    % Compute Pe using real exp/log instead of .^
    %    Effm_pos.^sgn_m  →  exp(log(Effm_pos) .* sgn_m)
    Pe = Pm ./ exp(sgn_m .* log(Effm_pos));
    
    % Preallocate I_bus and only compute where V_bus > 1
    I_bus = zeros(size(Pe));
    mask  = V_bus > 1;
    I_bus(mask) = Pe(mask) ./ V_bus(mask);
end

== matlab function simulink/Vehicle/Longitudinal Dynamics/Electric Motor Drive/Electric Motor/MATLAB Function1 ==
  data: input_torque input; corrected_torque output
function corrected_torque = fcn(input_torque)

    if input_torque < 0
        input_torque = input_torque  * -1;
    end
    corrected_torque = input_torque;

end

== matlab function simulink/Vehicle/Longitudinal Dynamics/Electric Motor Drive/Inverter/MATLAB Function ==
  data: V_bat input; V_bus output; Eff_I input; I_bus input; I_bat output
function [V_bus, I_bat]= fcn(V_bat, Eff_I, I_bus)
    
    V_bus = V_bat; % Vbus = Vbat * r, where r is the inverter conversion ratio % * I_bat * Eff_I^(sgn_Pbat))/I_bus;
    P_bus = V_bus * I_bus;
    sgn_Pbus = (P_bus + 10^-7)/(abs(P_bus) + 10^-7) + 0.001;

    if V_bat > 1
        I_bat = (P_bus / Eff_I^sgn_Pbus) / V_bat;
    else
        I_bat = 0;
    end
end

== matlab function simulink/Vehicle/Longitudinal Dynamics/Wheel/Drag Force ==
  data: Fdrag output; C_rr input; C_d input; v input; m input; A input
function Fdrag = drag_force(C_rr, C_d, v, m, A)
    g   = 9.81;             % gravity [m/s^2]
    rho = 1.225;            % air density [kg/m^3]

    F_roll   = C_rr * m * g;
    F_aero   = 0.5 * rho * C_d * A * v.^2;

    Fdrag = F_roll + F_aero;
end

== matlab function simulink/Vehicle/Longitudinal Dynamics/Brake System/MATLAB Function ==
  data: BBcmd input; Tb output; Tbcap input; w_wheel input
function Tb = fcn(BBcmd, Tbcap, w_wheel)
    Tb = BBcmd * Tbcap * (w_wheel / (abs(w_wheel) + 0.1));
end

== matlab function simulink/Vehicle/Lateral Dynamics/Tire Slip ==
  data: vy input; alpha_f output; vx input; steering_angle input; omega input; alpha_r output
function [alpha_f, alpha_r] = tire_slip(vy, vx, steering_angle, omega)
% tire_slip  Compute front/rear slip angles for the bicycle model
% Outputs: front and rear tire slip angle (rad)

  a = 1.2;
  b = 1.6;

  alpha_f = steering_angle - atan2(vy + a*omega, vx);
  alpha_r = -atan2(vy - b*omega, vx);
end

== matlab function simulink/Vehicle/Car Frame to Track Frame/Transformation//Rotation Function ==
  data: vx input; Xdot output; vy input; psi input; Ydot output
function [Xdot, Ydot] = fcn(vx, vy, psi)
    cosPsi = cos(psi);
    sinPsi = sin(psi);
    Xdot = cosPsi * vx - sinPsi * vy;
    Ydot = sinPsi * vx + cosPsi * vy;
end

== matlab function simulink/Vehicle/Lateral Dynamics/Tire Forces ==
  data: alpha_f input; Fyt output; alpha_r input; Fyr output
function [Fyt, Fyr] = tire_forces(alpha_f, alpha_r)
% tire_forces  Linear tire model for lateral force vs. slip angle
% determine front and rear tire tractice forces

  % cornering stiffnesses
  Cf = 8e4;
  Cr = 8e4;   

  % linear approximation
  Fyt = -Cf * alpha_f;
  Fyr = -Cr * alpha_r;
end

== matlab function simulink/Vehicle/Lateral Dynamics/MATLAB Function2 ==
  data: Fyt input; ay output; Fyr input; vx input; omega input; omega_dot output; m input; I input
function [ay, omega_dot] = LateralDynamics(Fyt, Fyr, vx, omega, m, I)
% LateralDynamics  Compute lateral and yaw accelerations
  ay        = (Fyt + Fyr)/m - vx * omega;
  omega_dot = (Fyt - Fyr)/I;
end

== matlab function simulink/Vehicle/Longitudinal Dynamics/Vehicle/MATLAB Function ==
  data: M input; a output; Fw input; Fd input; Fb input; I_rot input; r input; Vy input; Omega input; grade input
function a = vehicle(M, Fw, Fd, Fb, I_rot, r, Vy, Omega, grade)
% VEHICLE  Compute longitudinal acceleration including rotational inertia

    g = 9.81;  

    % convert rotational inertia to equivalent mass
    M_equiv = I_rot / r^2 + 0.1;  
    
    % gravitational component along grade
    Fg = M * g * sin(atan(grade));  
    
    % net longitudinal acceleration
    a = (Fw - Fd - Fb - Fg) / (M + M_equiv + 0.1) + Vy * Omega;
end

== matlab function simulink/Driver/track location ==
  data: x input; target_velocity output; v_des_turn input; v_des_straight input
function target_velocity = fcn(x, v_des_turn, v_des_straight)
if x >= 900 || x <= 0
    target_velocity = v_des_turn;
else
    target_velocity = v_des_straight;
end

== matlab function simulink/Environment/MATLAB Function ==
  data: x input; gradePct output; y input; height output
function [gradePct, height] = get_grade_function(x, y)
    % initialize the outputs
    height   = zeros(size(x));
    gradePct = zeros(size(x));

    % determine the segment types
    isBottom   = (x >=   0) & (x <= 900) & (y >=  -7.5) & (y <=   7.5);
    isTop      = (x >=   0) & (x <= 900) & (y >= 392.5) & (y <= 407.5);
    isStraight = isBottom | isTop;

    % determine height according to the equation
    xs = x(isStraight);
    t  = (xs - 450) ./ 50;
    L  = exp(t) ./ (1 + exp(t));
    height(isStraight) = 10 * L;

    % first turn height should be at 10
    isFirstTurn = (x > 900);
    height(isFirstTurn) = 10;

    % calculate the grade percent for the straights because it is zero on
    % the turns
    dhdx = 10 * (1/50) * (L .* (1 - L));
    gradePct(isStraight) = dhdx * 100;
end
